simulink model "First_Mask_ex"  (R2022b)
settings: Solver=VariableStepAuto  StartTime=0.0  StopTime=10.0  RelTol=1e-3
settings Model: Creator=Abanob_Sameh  LastModifiedBy=Abanob_Sameh

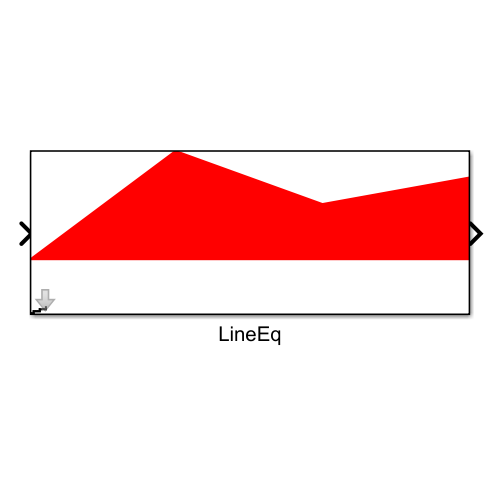
[thumbnail: Simulink's stored preview of the top-level diagram]
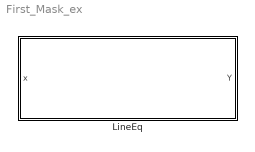
== system First_Mask_ex ==
  LineEq : Subsystem  mask{m=0, b=0}
      mask prompts: m "slope"; b "intersection"
      mask DialogControl DescGroupVar Prompt: Line eq Block
      mask Display:
      | x=linspace(0,1,101);
      | t=linspace(0,1,101);
      | plot(x,t);
      | patch([0 10 20 30 30 0], [10 30 20 25 10 10], [1 0 0]);

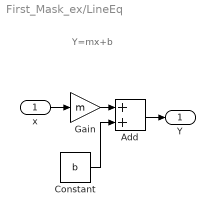
== system First_Mask_ex/LineEq ==
  note: Y=mx+b
  x : Inport
  Add : Sum
  Constant : Constant  Value=b
  Gain : Gain  Gain=m
  Y : Outport
  wires:
  Gain/1 -> Add/1
  Add/1 -> Y/1
  Constant/1 -> Add/2
  x/1 -> Gain/1
